simulink model "pid_nn"  (R2024b)
settings: Solver=VariableStepAuto  StartTime=0.0  StopTime=10.0  RelTol=1e-3
libraries: deeplib x1
settings Model: Creator=Pin Chuen  LastModifiedBy=Pin Chuen
settings DebuggingCC: UnderSpecifiedDimensionMsg=warning

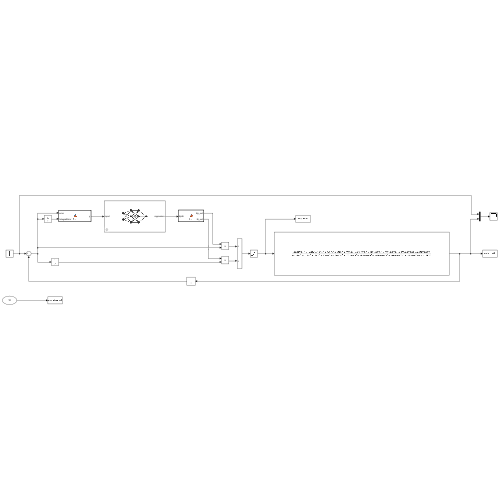
[thumbnail: Simulink's stored preview of the top-level diagram]
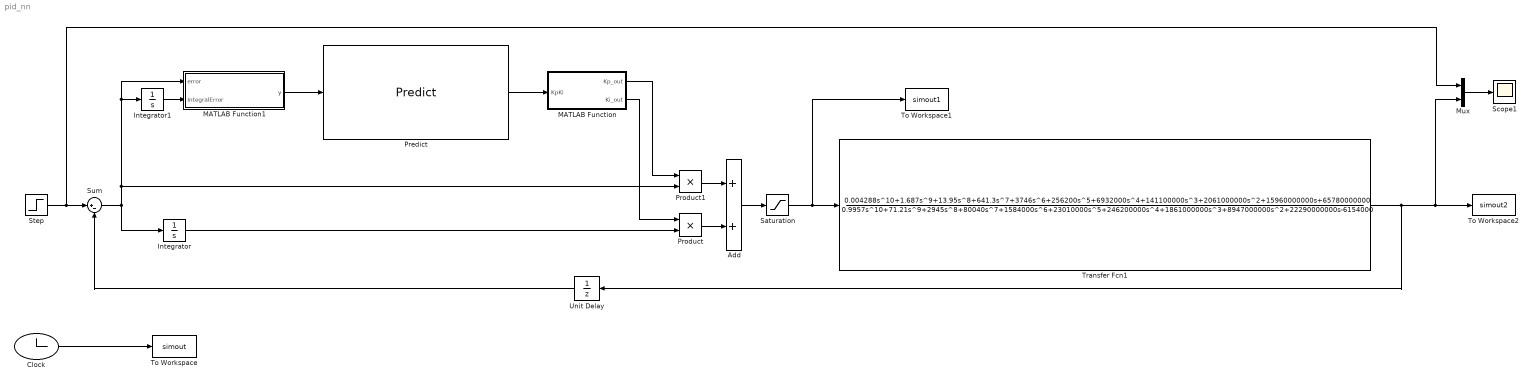
== system pid_nn ==
  Add : Sum
  Clock : Clock
  Integrator : Integrator
  Integrator1 : Integrator
  MATLAB Function : MATLAB Function  TreatAsAtomicUnit=on
  MATLAB Function1 : MATLAB Function  TreatAsAtomicUnit=on
  Mux : Mux  Inputs=2
  Predict : deeplib/Predict  Network=Network from MAT-file  NetworkFunction=squeezenet  NetworkFilePath=D:\UserDATA\Desktop\New folder\pid_nn_model3.mat  MiniBatchSize=128  InputDataFormats={'',''}  Predictions=on  Activations={}  ForceInterpretedSim=off  EnableDLNetwork=on  LastKnownNetworkFilePath=''  LastKnownNetworkTimeStamp=''
  Product : Product
  Product1 : Product
  Saturation : Saturate  UpperLimit=60  LowerLimit=-60
  Scope1 : Scope
  Step : Step  Before=50  After=50  SampleTime=0
  Sum : Sum  Inputs=|+-
  To Workspace : ToWorkspace  VariableName=simout  SampleTime=-1
      settings: Save2DSignal=2-D array (concatenate along first dimension)
  To Workspace1 : ToWorkspace  VariableName=simout1  SampleTime=-1
      settings: Save2DSignal=2-D array (concatenate along first dimension)
  To Workspace2 : ToWorkspace  VariableName=simout2  SampleTime=-1
      settings: Save2DSignal=2-D array (concatenate along first dimension)
  Transfer Fcn1 : TransferFcn  Numerator=[0.004288 1.687 13.95 641.3 3746 256200 6932000 141100000 2061000000 15960000000 65780000000]  Denominator=[0.9957 71.21 2945 80040 1584000 23010000 246200000 1861000000 8947000000 22290000000 -6154000]
  Unit Delay : UnitDelay  SampleTime=-1  HasFrameUpgradeWarning=on
  wires:
  Transfer Fcn1/1 -> To Workspace2/1, Mux/2, Unit Delay/1
  Step/1 -> Mux/1, Sum/1
  Saturation/1 -> To Workspace1/1, Transfer Fcn1/1
  Integrator/1 -> Product/2
  Product1/1 -> Add/1
  Product/1 -> Add/2
  MATLAB Function1/1(y) -> Predict/1
  Sum/1 -> MATLAB Function1/1(error), Integrator1/1, Product1/2, Integrator/1
  Integrator1/1 -> MATLAB Function1/2(IntegralError)
  Predict/1 -> MATLAB Function/1(KpKi)
  Mux/1 -> Scope1/1
  Add/1 -> Saturation/1
  MATLAB Function/1(Kp_out) -> Product1/1
  MATLAB Function/2(Ki_out) -> Product/1
  Unit Delay/1 -> Sum/2
  Clock/1 -> To Workspace/1

== matlab function pid_nn/MATLAB Function1 ==
  data: error input; y output; IntegralError input
function y = fcn(error, IntegralError)
    y = [error, IntegralError];
end

== matlab function pid_nn/MATLAB Function ==
  data: KpKi input; Kp_out output; Ki_out output
function [Kp_out, Ki_out] = fcn(KpKi)
    Kp_out = max(KpKi);  
    Ki_out = min(KpKi); 
end
